simulink model "UCT_PLab"  (R2018a)
settings: Solver=VariableStepAuto  StartTime=0.0  StopTime=0.1  RelTol=1e-3
undefined symbols (not defined in the file or in its folder): DiscIntNeverNeededParam
libraries: powerlib x98
settings Model: Creator=user  LastModifiedBy=user

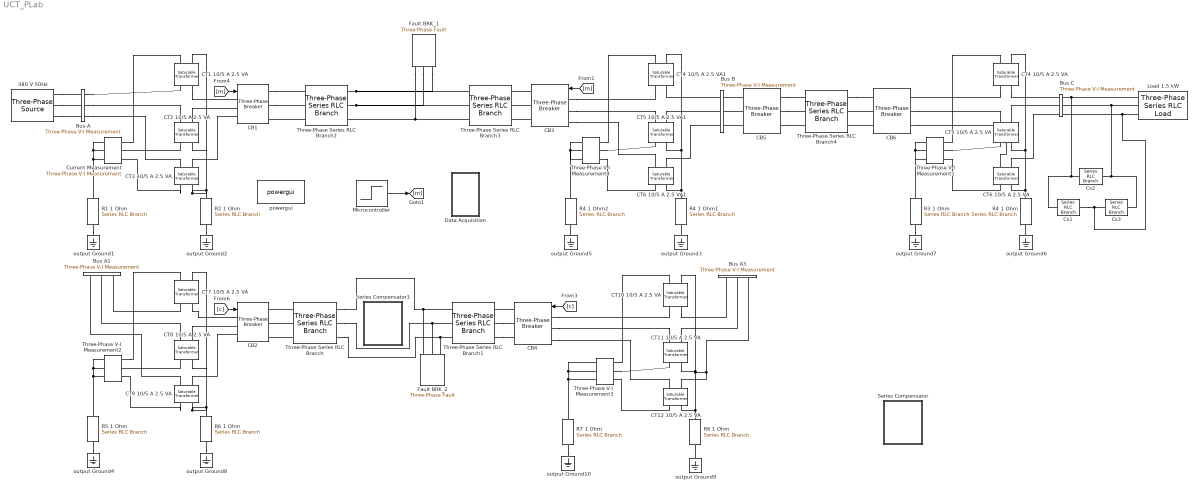
== system UCT_PLab ==
  380 V 50Hz : powerlib/Electrical Sources/Three-Phase Source  InternalConnection=Yg  VoltagePhases=off  Voltage=380  PhaseAngle=0  Voltage_phases=[25e3 25e3 25e3]/sqrt(3)  PhaseAngles_phases=[0 -120 +120]  Frequency=50  NonIdealSource=on  SpecifyImpedance=on  Resistance=132^2/30000/10  Inductance=132^2/30000/377  ShortCircuitLevel=15e3  BaseVoltage=380  XRratio=10  BusType=swing  Pref=150e6  Qref=0  Prefabc=[10e3, 10e3, 10e3]  Qrefabc=[0, 0, 0]  Qmin=0  Qmax=5e6
  Bus A : powerlib/Measurements/Three-Phase V-I Measurement  VoltageMeasurement=phase-to-phase  SetLabelV=on  LabelV=Vabc_B1  Vpu=off  VpuLL=on  CurrentMeasurement=yes  SetLabelI=on  LabelI=Iabc_B1  Ipu=off  Pbase=100e6  Vbase=380  OutputType=Complex  PhasorSimulation=off  PSBequivalent=0
  Bus A1 : powerlib/Measurements/Three-Phase V-I Measurement  VoltageMeasurement=no  SetLabelV=on  LabelV=Vabc_B1  Vpu=off  VpuLL=on  CurrentMeasurement=no  SetLabelI=on  LabelI=Iabc_B1  Ipu=off  Pbase=100e6  Vbase=380  OutputType=Complex  PhasorSimulation=off  PSBequivalent=0
  Bus A3 : powerlib/Measurements/Three-Phase V-I Measurement  VoltageMeasurement=no  SetLabelV=on  LabelV=Vabc_B1  Vpu=off  VpuLL=on  CurrentMeasurement=no  SetLabelI=on  LabelI=Iabc_B1  Ipu=off  Pbase=100e6  Vbase=380  OutputType=Complex  PhasorSimulation=off  PSBequivalent=0
  Bus B : powerlib/Measurements/Three-Phase V-I Measurement  VoltageMeasurement=phase-to-phase  SetLabelV=on  LabelV=Vabc_B2  Vpu=off  VpuLL=on  CurrentMeasurement=yes  SetLabelI=on  LabelI=Iabc_B2  Ipu=off  Pbase=100e6  Vbase=380  OutputType=Complex  PhasorSimulation=off  PSBequivalent=0
  Bus C : powerlib/Measurements/Three-Phase V-I Measurement  VoltageMeasurement=no  SetLabelV=on  LabelV=Vabc_B3  Vpu=off  VpuLL=on  CurrentMeasurement=no  SetLabelI=on  LabelI=Iabc_B3  Ipu=off  Pbase=100e6  Vbase=380  OutputType=Complex  PhasorSimulation=off  PSBequivalent=0
  CB1 : powerlib/Elements/Three-Phase Breaker  InitialState=closed  SwitchA=off  SwitchB=off  SwitchC=off  SwitchTimes=[5/60]  External=on  BreakerResistance=0.001  SnubberResistance=10e6  SnubberCapacitance=inf  Measurements=None
      settings: AttributesFormatString=\n
  CB2 : powerlib/Elements/Three-Phase Breaker  InitialState=open  SwitchA=on  SwitchB=on  SwitchC=on  SwitchTimes=[5/60]  External=on  BreakerResistance=0.001  SnubberResistance=1000e6  SnubberCapacitance=inf  Measurements=None
      settings: AttributesFormatString=\n
  CB3 : powerlib/Elements/Three-Phase Breaker  InitialState=closed  SwitchA=off  SwitchB=off  SwitchC=off  SwitchTimes=[5/60]  External=on  BreakerResistance=0.001  SnubberResistance=10e6  SnubberCapacitance=inf  Measurements=None
      settings: AttributesFormatString=\n
  CB4 : powerlib/Elements/Three-Phase Breaker  InitialState=open  SwitchA=off  SwitchB=off  SwitchC=off  SwitchTimes=[5/60]  External=on  BreakerResistance=0.001  SnubberResistance=1000e6  SnubberCapacitance=inf  Measurements=None
      settings: AttributesFormatString=\n
  CB5 : powerlib/Elements/Three-Phase Breaker  InitialState=closed  SwitchA=off  SwitchB=off  SwitchC=off  SwitchTimes=[1/60]  External=off  BreakerResistance=0.001  SnubberResistance=10e6  SnubberCapacitance=inf  Measurements=None
      settings: AttributesFormatString=\n
  CB6 : powerlib/Elements/Three-Phase Breaker  InitialState=closed  SwitchA=off  SwitchB=off  SwitchC=off  SwitchTimes=[1/60]  External=off  BreakerResistance=0.001  SnubberResistance=10e6  SnubberCapacitance=inf  Measurements=None
      settings: AttributesFormatString=\n
  CT1 10/5 A 2.5 VA : powerlib/Elements/Saturable Transformer  ThreeWindings=off  Hysteresis=off  DataFile='hysteresis'  Measurements=Winding currents  UNITS=pu  NominalPower=[2.5 50]  Winding1=[2.5*5/10 0.001 0.04]  Winding2=[5 0.001 0.04]  Winding3=[5 0.001 0.039999]  Saturation=[0 0 ; 0.01 10 ; 1 10.5]  CoreLoss=100  MoreParameters=off  BreakLoop=off  DataType=off  InitialFlux=-1.58250193491149e-05  TransfoNumber=1
      settings: AttributesFormatString=\n  SourceProductName=Simscape Power Systems  SourceProductBaseCode=PS
  CT10 10/5 A 2.5 VA : powerlib/Elements/Saturable Transformer  ThreeWindings=off  Hysteresis=off  DataFile='hysteresis'  Measurements=Winding currents  UNITS=pu  NominalPower=[15 50]  Winding1=[5*5/40 0.001 0.04]  Winding2=[5 0.001 0.04]  Winding3=[5 0.001 0.039999]  Saturation=[0 0 ; 0.01 10 ; 1 10.5]  CoreLoss=100  MoreParameters=off  BreakLoop=off  DataType=off  InitialFlux=0  TransfoNumber=1
      settings: AttributesFormatString=\n  SourceProductName=Simscape Power Systems  SourceProductBaseCode=PS
  CT11 10/5 A 2.5 VA : powerlib/Elements/Saturable Transformer  ThreeWindings=off  Hysteresis=off  DataFile='hysteresis'  Measurements=Winding currents  UNITS=pu  NominalPower=[15 50]  Winding1=[5*5/40 0.001 0.04]  Winding2=[5 0.001 0.04 ]  Winding3=[5 0.001 0.04 ]  Saturation=[0 0 ; 0.01 10 ; 1 10.5]  CoreLoss=100  MoreParameters=off  BreakLoop=off  DataType=off  InitialFlux=0  TransfoNumber=1
      settings: AttributesFormatString=\n  SourceProductName=Simscape Power Systems  SourceProductBaseCode=PS
  CT12 10/5 A 2.5 VA : powerlib/Elements/Saturable Transformer  ThreeWindings=off  Hysteresis=off  DataFile='hysteresis'  Measurements=Winding currents  UNITS=pu  NominalPower=[15 50]  Winding1=[5*5/40 0.001 0.04]  Winding2=[5 0.001 0.04]  Winding3=[5 0.001 0.039999]  Saturation=[0 0 ; 0.01 10 ; 1 10.5]  CoreLoss=100  MoreParameters=off  BreakLoop=off  DataType=off  InitialFlux=0  TransfoNumber=1
      settings: AttributesFormatString=\n  SourceProductName=Simscape Power Systems  SourceProductBaseCode=PS
  CT2 10/5 A 2.5 VA : powerlib/Elements/Saturable Transformer  ThreeWindings=off  Hysteresis=off  DataFile='hysteresis'  Measurements=Winding currents  UNITS=pu  NominalPower=[2.5 50]  Winding1=[2.5*5/10 0.001 0.04]  Winding2=[5 0.001 0.04 ]  Winding3=[5 0.001 0.04 ]  Saturation=[0 0 ; 0.01 10 ; 1 10.5]  CoreLoss=100  MoreParameters=off  BreakLoop=off  DataType=off  InitialFlux=5.84628665097414e-06  TransfoNumber=1
      settings: AttributesFormatString=\n  SourceProductName=Simscape Power Systems  SourceProductBaseCode=PS
  CT3 10/5 A 2.5 VA : powerlib/Elements/Saturable Transformer  ThreeWindings=off  Hysteresis=off  DataFile='hysteresis'  Measurements=Winding currents  UNITS=pu  NominalPower=[2.5 50]  Winding1=[2.5*5/10 0.001 0.04]  Winding2=[5 0.001 0.04]  Winding3=[5 0.001 0.039999]  Saturation=[0 0 ; 0.01 10 ; 1 10.5]  CoreLoss=100  MoreParameters=off  BreakLoop=off  DataType=off  InitialFlux=9.97873269594806e-06  TransfoNumber=1
      settings: AttributesFormatString=\n  SourceProductName=Simscape Power Systems  SourceProductBaseCode=PS
  CT4 10/5 A 2.5 VA : powerlib/Elements/Saturable Transformer  ThreeWindings=off  Hysteresis=off  DataFile='hysteresis'  Measurements=Winding currents  UNITS=pu  NominalPower=[2.5 50]  Winding1=[2.5*5/10 0.001 0.04]  Winding2=[5 0.001 0.04]  Winding3=[5 0.001 0.039999]  Saturation=[0 0 ; 0.01 10 ; 1 10.5]  CoreLoss=100  MoreParameters=off  BreakLoop=off  DataType=off  InitialFlux=-1.58243299206724e-05  TransfoNumber=1
      settings: AttributesFormatString=\n  SourceProductName=Simscape Power Systems  SourceProductBaseCode=PS
  CT4 10/5 A 2.5 VA1 : powerlib/Elements/Saturable Transformer  ThreeWindings=off  Hysteresis=off  DataFile='hysteresis'  Measurements=Winding currents  UNITS=pu  NominalPower=[2.5 50]  Winding1=[2.5*5/10 0.001 0.04]  Winding2=[5 0.001 0.04]  Winding3=[5 0.001 0.039999]  Saturation=[0 0 ; 0.01 10 ; 1 10.5]  CoreLoss=100  MoreParameters=off  BreakLoop=off  DataType=off  InitialFlux=-1.58243299202559e-05  TransfoNumber=1
      link override Model/1-D Lookup Table: NumberOfTableDimensions=1
      settings: AttributesFormatString=\n  SourceProductName=Simscape Power Systems  SourceProductBaseCode=PS
  CT5 10/5 A 2.5 VA : powerlib/Elements/Saturable Transformer  ThreeWindings=off  Hysteresis=off  DataFile='hysteresis'  Measurements=Winding currents  UNITS=pu  NominalPower=[2.5 50]  Winding1=[2.5*5/10 0.001 0.04]  Winding2=[5 0.001 0.04 ]  Winding3=[5 0.001 0.04 ]  Saturation=[0 0 ; 0.01 10 ; 1 10.5]  CoreLoss=100  MoreParameters=off  BreakLoop=off  DataType=off  InitialFlux=5.86672769127917e-06  TransfoNumber=1
      settings: AttributesFormatString=\n  SourceProductName=Simscape Power Systems  SourceProductBaseCode=PS
  CT5 10/5 A 2.5 VA1 : powerlib/Elements/Saturable Transformer  ThreeWindings=off  Hysteresis=off  DataFile='hysteresis'  Measurements=Winding currents  UNITS=pu  NominalPower=[2.5 50]  Winding1=[2.5*5/10 0.001 0.04]  Winding2=[5 0.001 0.04 ]  Winding3=[5 0.001 0.04 ]  Saturation=[0 0 ; 0.01 10 ; 1 10.5]  CoreLoss=100  MoreParameters=off  BreakLoop=off  DataType=off  InitialFlux=5.86672769116839e-06  TransfoNumber=1
      settings: AttributesFormatString=\n  SourceProductName=Simscape Power Systems  SourceProductBaseCode=PS
  CT6 10/5 A 2.5 VA : powerlib/Elements/Saturable Transformer  ThreeWindings=off  Hysteresis=off  DataFile='hysteresis'  Measurements=Winding currents  UNITS=pu  NominalPower=[2.5 50]  Winding1=[2.5*5/10 0.001 0.04]  Winding2=[5 0.001 0.04]  Winding3=[5 0.001 0.039999]  Saturation=[0 0 ; 0.01 10 ; 1 10.5]  CoreLoss=100  MoreParameters=off  BreakLoop=off  DataType=off  InitialFlux=9.95760222411303e-06  TransfoNumber=1
      settings: AttributesFormatString=\n  SourceProductName=Simscape Power Systems  SourceProductBaseCode=PS
  CT6 10/5 A 2.5 VA1 : powerlib/Elements/Saturable Transformer  ThreeWindings=off  Hysteresis=off  DataFile='hysteresis'  Measurements=Winding currents  UNITS=pu  NominalPower=[2.5 50]  Winding1=[2.5*5/10 0.001 0.04]  Winding2=[5 0.001 0.04]  Winding3=[5 0.001 0.039999]  Saturation=[0 0 ; 0.01 10 ; 1 10.5]  CoreLoss=100  MoreParameters=off  BreakLoop=off  DataType=off  InitialFlux=9.95760222411131e-06  TransfoNumber=1
      settings: AttributesFormatString=\n  SourceProductName=Simscape Power Systems  SourceProductBaseCode=PS
  CT7 10/5 A 2.5 VA : powerlib/Elements/Saturable Transformer  ThreeWindings=off  Hysteresis=off  DataFile='hysteresis'  Measurements=Winding currents  UNITS=pu  NominalPower=[15 50]  Winding1=[5*1/600 0.001 0.04]  Winding2=[5*5/40 0.001 0.04]  Winding3=[5 0.001 0.039999]  Saturation=[0 0 ; 0.01 10 ; 1 10.5]  CoreLoss=100  MoreParameters=off  BreakLoop=off  DataType=off  InitialFlux=0  TransfoNumber=1
      settings: AttributesFormatString=\n  SourceProductName=Simscape Power Systems  SourceProductBaseCode=PS
  CT8 10/5 A 2.5 VA : powerlib/Elements/Saturable Transformer  ThreeWindings=off  Hysteresis=off  DataFile='hysteresis'  Measurements=Winding currents  UNITS=pu  NominalPower=[15 50]  Winding1=[5*5/40 0.001 0.04]  Winding2=[5 0.001 0.04 ]  Winding3=[5 0.001 0.04 ]  Saturation=[0 0 ; 0.01 10 ; 1 10.5]  CoreLoss=100  MoreParameters=off  BreakLoop=off  DataType=off  InitialFlux=0  TransfoNumber=1
      settings: AttributesFormatString=\n  SourceProductName=Simscape Power Systems  SourceProductBaseCode=PS
  CT9 10/5 A 2.5 VA : powerlib/Elements/Saturable Transformer  ThreeWindings=off  Hysteresis=off  DataFile='hysteresis'  Measurements=Winding currents  UNITS=pu  NominalPower=[15 50]  Winding1=[5*5/40 0.001 0.04]  Winding2=[5 0.001 0.04]  Winding3=[5 0.001 0.039999]  Saturation=[0 0 ; 0.01 10 ; 1 10.5]  CoreLoss=100  MoreParameters=off  BreakLoop=off  DataType=off  InitialFlux=0  TransfoNumber=1
      settings: AttributesFormatString=\n  SourceProductName=Simscape Power Systems  SourceProductBaseCode=PS
  Cs1 : powerlib/Elements/Series RLC Branch  LConnTagsString=__new0  RConnTagsString=__new0  BranchType=C  Resistance=1.0  Inductance=1.0  SetiL0=off  InitialCurrent=0  Capacitance=2.0e-6  Setx0=off  InitialVoltage=0  Measurements=None
  Cs2 : powerlib/Elements/Series RLC Branch  LConnTagsString=__new0  RConnTagsString=__new0  BranchType=C  Resistance=1.0  Inductance=1.0  SetiL0=off  InitialCurrent=0  Capacitance=2.0e-6  Setx0=off  InitialVoltage=0  Measurements=None
  Cs3 : powerlib/Elements/Series RLC Branch  LConnTagsString=__new0  RConnTagsString=__new0  BranchType=C  Resistance=1.0  Inductance=1.0  SetiL0=off  InitialCurrent=0  Capacitance=2.0e-6  Setx0=off  InitialVoltage=0  Measurements=None
  Current Measurement : powerlib/Measurements/Three-Phase V-I Measurement  VoltageMeasurement=no  SetLabelV=off  LabelV=Vabc  Vpu=off  VpuLL=off  CurrentMeasurement=yes  SetLabelI=on  LabelI=Iabc  Ipu=off  Pbase=100e6  Vbase=500e3  OutputType=Complex  PhasorSimulation=off  PSBequivalent=0
  Data Acquisition : Subsystem  mask(Data Acquisition){}
      mask Display: disp('Scopes')
  Fault BRK_1 : powerlib/Elements/Three-Phase Fault  InitialStates=0  FaultA=on  FaultB=on  FaultC=on  GroundFault=on  SwitchTimes=[1/60 ]  External=off  SwitchStatus=NaN  FaultResistance=0.0001  GroundResistance=10  SnubberResistance=1e6  SnubberCapacitance=inf  Measurements=Fault currents
  Fault BRK_2 : powerlib/Elements/Three-Phase Fault  InitialStates=0  FaultA=off  FaultB=off  FaultC=off  GroundFault=off  SwitchTimes=[1/60 8/60]  External=off  SwitchStatus=NaN  FaultResistance=0.001  GroundResistance=0.01  SnubberResistance=1e6  SnubberCapacitance=inf  Measurements=Fault currents
  Load 1.5 kW : powerlib/Elements/Three-Phase Series RLC Load  LConnTagsString=A|B|C  Configuration=Y (grounded)  NominalVoltage=380  Vabc=[1e3 1e3 1e3]  Vabcp=[1e3 1e3 1e3]  NominalFrequency=50  UnbalancedPower=off  ActivePower=16.85  InductivePower=95.05  CapacitivePower=0  Pabc=[10e3 9e3 11e3]  QLabc=[100 90 110]  QCabc=[100 90 110]  Pabcp=[10e3 9e3 11e3]  QLabcp=[100 90 110]  QCabcp=[100 90 110]  Measurements=None  LoadType=constant Z
  Microcontroller : Step  Time=4/60  Before=1  VectorParams1D=off  ZeroCross=off
  R1 1 Ohm : powerlib/Elements/Series RLC Branch  LConnTagsString=__new0  RConnTagsString=__new0  BranchType=R  Resistance=1  Inductance=[]  SetiL0=off  InitialCurrent=0  Capacitance=[]  Setx0=off  InitialVoltage=0  Measurements=None
  R2 1 Ohm : powerlib/Elements/Series RLC Branch  LConnTagsString=__new0  RConnTagsString=__new0  BranchType=R  Resistance=1  Inductance=[]  SetiL0=off  InitialCurrent=0  Capacitance=[]  Setx0=off  InitialVoltage=0  Measurements=None
  R3 1 Ohm : powerlib/Elements/Series RLC Branch  LConnTagsString=__new0  RConnTagsString=__new0  BranchType=R  Resistance=1  Inductance=[]  SetiL0=off  InitialCurrent=0  Capacitance=[]  Setx0=off  InitialVoltage=0  Measurements=None
  R4 1 Ohm : powerlib/Elements/Series RLC Branch  LConnTagsString=__new0  RConnTagsString=__new0  BranchType=R  Resistance=1  Inductance=[]  SetiL0=off  InitialCurrent=0  Capacitance=[]  Setx0=off  InitialVoltage=0  Measurements=None
  R4 1 Ohm1 : powerlib/Elements/Series RLC Branch  LConnTagsString=__new0  RConnTagsString=__new0  BranchType=R  Resistance=1  Inductance=[]  SetiL0=off  InitialCurrent=0  Capacitance=[]  Setx0=off  InitialVoltage=0  Measurements=None
  R4 1 Ohm2 : powerlib/Elements/Series RLC Branch  LConnTagsString=__new0  RConnTagsString=__new0  BranchType=R  Resistance=1  Inductance=[]  SetiL0=off  InitialCurrent=0  Capacitance=[]  Setx0=off  InitialVoltage=0  Measurements=None
  R5 1 Ohm : powerlib/Elements/Series RLC Branch  LConnTagsString=__new0  RConnTagsString=__new0  BranchType=R  Resistance=1  Inductance=[]  SetiL0=off  InitialCurrent=0  Capacitance=[]  Setx0=off  InitialVoltage=0  Measurements=None
  R6 1 Ohm : powerlib/Elements/Series RLC Branch  LConnTagsString=__new0  RConnTagsString=__new0  BranchType=R  Resistance=1  Inductance=[]  SetiL0=off  InitialCurrent=0  Capacitance=[]  Setx0=off  InitialVoltage=0  Measurements=None
  R7 1 Ohm : powerlib/Elements/Series RLC Branch  LConnTagsString=__new0  RConnTagsString=__new0  BranchType=R  Resistance=1  Inductance=[]  SetiL0=off  InitialCurrent=0  Capacitance=[]  Setx0=off  InitialVoltage=0  Measurements=None
  R8 1 Ohm : powerlib/Elements/Series RLC Branch  LConnTagsString=__new0  RConnTagsString=__new0  BranchType=R  Resistance=1  Inductance=[]  SetiL0=off  InitialCurrent=0  Capacitance=[]  Setx0=off  InitialVoltage=0  Measurements=None
  Series Compensator : Subsystem
      mask Display: plot(0,0,100,100,[25 45],[50 50], [45 45],[35 65],[55 55],[35 65], [55 75],[50 50])
  Series Compensator1 : Subsystem
      mask Display: plot(0,0,100,100,[25 45],[50 50], [45 45],[35 65],[55 55],[35 65], [55 75],[50 50])
  Three-Phase Series RLC Branch : powerlib/Elements/Three-Phase Series RLC Branch  LConnTagsString=A|B|C  RConnTagsString=A|B|C  BranchType=RL  Resistance=1.60  Inductance=6.47e-3  Capacitance=0  Measurements=None
  Three-Phase Series RLC Branch1 : powerlib/Elements/Three-Phase Series RLC Branch  LConnTagsString=A|B|C  RConnTagsString=A|B|C  BranchType=RL  Resistance=1.60  Inductance=6.47e-3  Capacitance=0  Measurements=None
  Three-Phase Series RLC Branch2 : powerlib/Elements/Three-Phase Series RLC Branch  LConnTagsString=A|B|C  RConnTagsString=A|B|C  BranchType=RL  Resistance=1.60  Inductance=106.47e-3  Capacitance=0  Measurements=None
  Three-Phase Series RLC Branch3 : powerlib/Elements/Three-Phase Series RLC Branch  LConnTagsString=A|B|C  RConnTagsString=A|B|C  BranchType=RL  Resistance=1.60  Inductance=6.47e-3  Capacitance=0  Measurements=None
  Three-Phase Series RLC Branch4 : powerlib/Elements/Three-Phase Series RLC Branch  LConnTagsString=A|B|C  RConnTagsString=A|B|C  BranchType=RL  Resistance=1.35  Inductance=7.25e-3  Capacitance=0  Measurements=None
  Three-Phase V-I Measurement1 : powerlib/Measurements/Three-Phase V-I Measurement  VoltageMeasurement=no  SetLabelV=off  LabelV=Vabc  Vpu=off  VpuLL=off  CurrentMeasurement=yes  SetLabelI=on  LabelI=Iabc1  Ipu=off  Pbase=100e6  Vbase=500e3  OutputType=Complex  PhasorSimulation=off  PSBequivalent=0
  Three-Phase V-I Measurement2 : powerlib/Measurements/Three-Phase V-I Measurement  VoltageMeasurement=no  SetLabelV=off  LabelV=Vabc  Vpu=off  VpuLL=off  CurrentMeasurement=no  SetLabelI=on  LabelI=Iabc2  Ipu=off  Pbase=100e6  Vbase=500e3  OutputType=Complex  PhasorSimulation=off  PSBequivalent=0
  Three-Phase V-I Measurement3 : powerlib/Measurements/Three-Phase V-I Measurement  VoltageMeasurement=no  SetLabelV=off  LabelV=Vabc  Vpu=off  VpuLL=off  CurrentMeasurement=no  SetLabelI=on  LabelI=Iabc3  Ipu=off  Pbase=100e6  Vbase=500e3  OutputType=Complex  PhasorSimulation=off  PSBequivalent=0
  Three-Phase V-I Measurement4 : powerlib/Measurements/Three-Phase V-I Measurement  VoltageMeasurement=no  SetLabelV=off  LabelV=Vabc  Vpu=off  VpuLL=off  CurrentMeasurement=no  SetLabelI=on  LabelI=Iabc1  Ipu=off  Pbase=100e6  Vbase=500e3  OutputType=Complex  PhasorSimulation=off  PSBequivalent=0
  output Ground{1..10} (10 alike) : powerlib/Elements/Ground  LConnTagsString=a
  powergui : powerlib/powergui  Priority=2  SimulationMode=Discrete  SampleTime=50e-6  frequency=60  Iterations=50  frequencyindice=50  Pbase=100e6  ErrMax=0.0001  UnitsV=kV  UnitsW=MW  buscounter=0  FunctionMessages=off  echomessages=off  EnableUseOfTLC=off  CurrentSourceSwitches=off  DisableSnubberDevices=off  DisableRonSwitches=off  DisableVfSwitches=off  DisplayEquations=off  SolverType=Tustin/Backward Euler (TBE)  Interpol=off  ExternalGateDelay=off  methode=off  Ts=100  x0status=blocks  SPID=off  SwTol=0  HookPort=off  RestoreLinks=warning  ResistiveCurrentMeasurement=off  Frange=0:0.5:500  Ylog=off  Xlog=off  ShowGrid=off  save=on  variable=Zmes  structure=0  ZoomFFT=on  StartTime=0.0  cycles=1  DisplayStyle=off  fundamental=60  FreqAxis=off  MaxFrequency=1000  frequencyindicesteady=1  RmsSteady=1  display=off
  wires:
  Microcontroller/1 -> [m]
  [m] -> CB3/1
  [m] -> CB1/1
  [c] -> CB4/1
  [c] -> CB2/1
  connections:
  CT9 10/5 A 2.5 VA/LConn1 -- Bus A1/RConn3
  Bus A/RConn1 -- CT1 10/5 A 2.5 VA/LConn1
  Current Measurement/RConn3 -- R1 1 Ohm/LConn1 -- Current Measurement/RConn2 -- Current Measurement/RConn1
  Bus A/RConn2 -- CT2 10/5 A 2.5 VA/LConn1
  CT3 10/5 A 2.5 VA/RConn2 -- R2 1 Ohm/LConn1 -- CT1 10/5 A 2.5 VA/RConn2 -- CT2 10/5 A 2.5 VA/RConn2
  380 V 50Hz/RConn1 -- Bus A/LConn1
  380 V 50Hz/RConn3 -- Bus A/LConn3
  CB3/RConn3 -- Three-Phase Series RLC Branch3/RConn3
  CB1/RConn1 -- Three-Phase Series RLC Branch2/LConn1
  CB1/RConn2 -- Three-Phase Series RLC Branch2/LConn2
  CT3 10/5 A 2.5 VA/RConn1 -- Current Measurement/LConn3
  CB3/RConn2 -- Three-Phase Series RLC Branch3/RConn2
  CB3/RConn1 -- Three-Phase Series RLC Branch3/RConn1
  CT2 10/5 A 2.5 VA/LConn2 -- CB1/LConn2
  CB1/LConn3 -- CT3 10/5 A 2.5 VA/LConn2
  380 V 50Hz/RConn2 -- Bus A/LConn2
  CT1 10/5 A 2.5 VA/LConn2 -- CB1/LConn1
  Current Measurement/LConn1 -- CT1 10/5 A 2.5 VA/RConn1
  R2 1 Ohm/RConn1 -- output Ground2/LConn1
  R1 1 Ohm/RConn1 -- output Ground1/LConn1
  CT2 10/5 A 2.5 VA/RConn1 -- Current Measurement/LConn2
  CT9 10/5 A 2.5 VA/RConn2 -- R6 1 Ohm/LConn1 -- CT7 10/5 A 2.5 VA/RConn2 -- CT8 10/5 A 2.5 VA/RConn2
  Three-Phase V-I Measurement2/RConn3 -- Three-Phase V-I Measurement2/RConn1 -- Three-Phase V-I Measurement2/RConn2 -- R5 1 Ohm/LConn1
  Three-Phase Series RLC Branch/RConn1 -- Three-Phase Series RLC Branch1/LConn1 -- Fault BRK_2/LConn1
  Three-Phase Series RLC Branch/RConn2 -- Three-Phase Series RLC Branch1/LConn2 -- Fault BRK_2/LConn2
  Three-Phase Series RLC Branch/RConn3 -- Three-Phase Series RLC Branch1/LConn3 -- Fault BRK_2/LConn3
  R7 1 Ohm/LConn1 -- Three-Phase V-I Measurement3/RConn3 -- Three-Phase V-I Measurement3/RConn2 -- Three-Phase V-I Measurement3/RConn1
  Three-Phase Series RLC Branch1/RConn2 -- CB4/RConn2
  R5 1 Ohm/RConn1 -- output Ground4/LConn1
  CT8 10/5 A 2.5 VA/RConn1 -- Three-Phase V-I Measurement2/LConn2
  CT9 10/5 A 2.5 VA/RConn1 -- Three-Phase V-I Measurement2/LConn3
  CB4/LConn3 -- CT12 10/5 A 2.5 VA/LConn1
  CT7 10/5 A 2.5 VA/LConn2 -- CB2/LConn1
  CB2/LConn3 -- CT9 10/5 A 2.5 VA/LConn2
  output Ground9/LConn1 -- R8 1 Ohm/RConn1
  Three-Phase Series RLC Branch1/RConn3 -- CB4/RConn3
  R7 1 Ohm/RConn1 -- output Ground10/LConn1
  CT8 10/5 A 2.5 VA/LConn2 -- CB2/LConn2
  Three-Phase V-I Measurement2/LConn1 -- CT7 10/5 A 2.5 VA/RConn1
  Three-Phase Series RLC Branch/LConn1 -- CB2/RConn1
  R6 1 Ohm/RConn1 -- output Ground8/LConn1
  Three-Phase V-I Measurement3/LConn2 -- CT11 10/5 A 2.5 VA/RConn1
  Three-Phase Series RLC Branch/LConn2 -- CB2/RConn2
  Three-Phase Series RLC Branch/LConn3 -- CB2/RConn3
  CB4/RConn1 -- Three-Phase Series RLC Branch1/RConn1
  CB4/LConn2 -- CT11 10/5 A 2.5 VA/LConn1
  Three-Phase V-I Measurement3/LConn1 -- CT10 10/5 A 2.5 VA/RConn1
  CB4/LConn1 -- CT10 10/5 A 2.5 VA/LConn1
  Three-Phase V-I Measurement3/LConn3 -- CT12 10/5 A 2.5 VA/RConn1
  CB6/RConn2 -- Three-Phase Series RLC Branch4/RConn2
  CB6/RConn3 -- Three-Phase Series RLC Branch4/RConn3
  Three-Phase Series RLC Branch4/RConn1 -- CB6/RConn1
  Cs1/RConn1 -- Bus C/RConn3 -- Load 1.5 kW/LConn3 -- Cs3/LConn1
  CB5/RConn3 -- Bus B/RConn3
  CB5/RConn1 -- Bus B/RConn1
  CB5/RConn2 -- Bus B/RConn2
  Three-Phase Series RLC Branch2/LConn3 -- CB1/RConn3
  CT8 10/5 A 2.5 VA/LConn1 -- Bus A1/RConn2
  CT7 10/5 A 2.5 VA/LConn1 -- Bus A1/RConn1
  CT11 10/5 A 2.5 VA/LConn2 -- Bus A3/RConn2
  CT10 10/5 A 2.5 VA/LConn2 -- Bus A3/RConn3
  CT11 10/5 A 2.5 VA/RConn2 -- Bus A3/RConn1 -- CT12 10/5 A 2.5 VA/LConn2 -- CT12 10/5 A 2.5 VA/RConn2 -- R8 1 Ohm/LConn1 -- CT10 10/5 A 2.5 VA/RConn2
  CB5/LConn3 -- Three-Phase Series RLC Branch4/LConn3
  CB5/LConn2 -- Three-Phase Series RLC Branch4/LConn2
  CB5/LConn1 -- Three-Phase Series RLC Branch4/LConn1
  Three-Phase Series RLC Branch2/RConn1 -- Three-Phase Series RLC Branch3/LConn1 -- Fault BRK_1/LConn1
  Three-Phase V-I Measurement1/RConn2 -- Three-Phase V-I Measurement1/RConn1 -- Three-Phase V-I Measurement1/RConn3 -- R3 1 Ohm/LConn1
  CT4 10/5 A 2.5 VA/RConn2 -- CT5 10/5 A 2.5 VA/RConn2 -- CT6 10/5 A 2.5 VA/RConn2 -- R4 1 Ohm/LConn1
  R3 1 Ohm/RConn1 -- output Ground7/LConn1
  Three-Phase V-I Measurement1/LConn2 -- CT5 10/5 A 2.5 VA/RConn1
  output Ground6/LConn1 -- R4 1 Ohm/RConn1
  CT5 10/5 A 2.5 VA/LConn2 -- Bus C/LConn2
  CB6/LConn2 -- CT5 10/5 A 2.5 VA/LConn1
  CT4 10/5 A 2.5 VA/LConn1 -- CB6/LConn1
  Three-Phase V-I Measurement1/LConn1 -- CT4 10/5 A 2.5 VA/RConn1
  CT4 10/5 A 2.5 VA/LConn2 -- Bus C/LConn1
  CB6/LConn3 -- CT6 10/5 A 2.5 VA/LConn1
  CT6 10/5 A 2.5 VA/LConn2 -- Bus C/LConn3
  Three-Phase V-I Measurement1/LConn3 -- CT6 10/5 A 2.5 VA/RConn1
  Three-Phase V-I Measurement4/RConn2 -- Three-Phase V-I Measurement4/RConn1 -- Three-Phase V-I Measurement4/RConn3 -- R4 1 Ohm2/LConn1
  CT4 10/5 A 2.5 VA1/RConn2 -- CT5 10/5 A 2.5 VA1/RConn2 -- CT6 10/5 A 2.5 VA1/RConn2 -- R4 1 Ohm1/LConn1
  CB3/LConn1 -- CT4 10/5 A 2.5 VA1/LConn1
  output Ground3/LConn1 -- R4 1 Ohm1/RConn1
  Three-Phase V-I Measurement4/LConn1 -- CT4 10/5 A 2.5 VA1/RConn1
  Three-Phase V-I Measurement4/LConn3 -- CT6 10/5 A 2.5 VA1/RConn1
  CT6 10/5 A 2.5 VA1/LConn2 -- Bus B/LConn3
  CB3/LConn3 -- CT6 10/5 A 2.5 VA1/LConn1
  Bus B/LConn1 -- CT4 10/5 A 2.5 VA1/LConn2
  Three-Phase V-I Measurement4/LConn2 -- CT5 10/5 A 2.5 VA1/RConn1
  Bus B/LConn2 -- CT5 10/5 A 2.5 VA1/LConn2
  output Ground5/LConn1 -- R4 1 Ohm2/RConn1
  CB3/LConn2 -- CT5 10/5 A 2.5 VA1/LConn1
  Bus A/RConn3 -- CT3 10/5 A 2.5 VA/LConn1
  Three-Phase Series RLC Branch2/RConn2 -- Three-Phase Series RLC Branch3/LConn2 -- Fault BRK_1/LConn2
  Fault BRK_1/LConn3 -- Three-Phase Series RLC Branch3/LConn3 -- Three-Phase Series RLC Branch2/RConn3
  Bus C/RConn2 -- Cs2/RConn1 -- Cs3/RConn1 -- Load 1.5 kW/LConn2
  Bus C/RConn1 -- Cs1/LConn1 -- Cs2/LConn1 -- Load 1.5 kW/LConn1

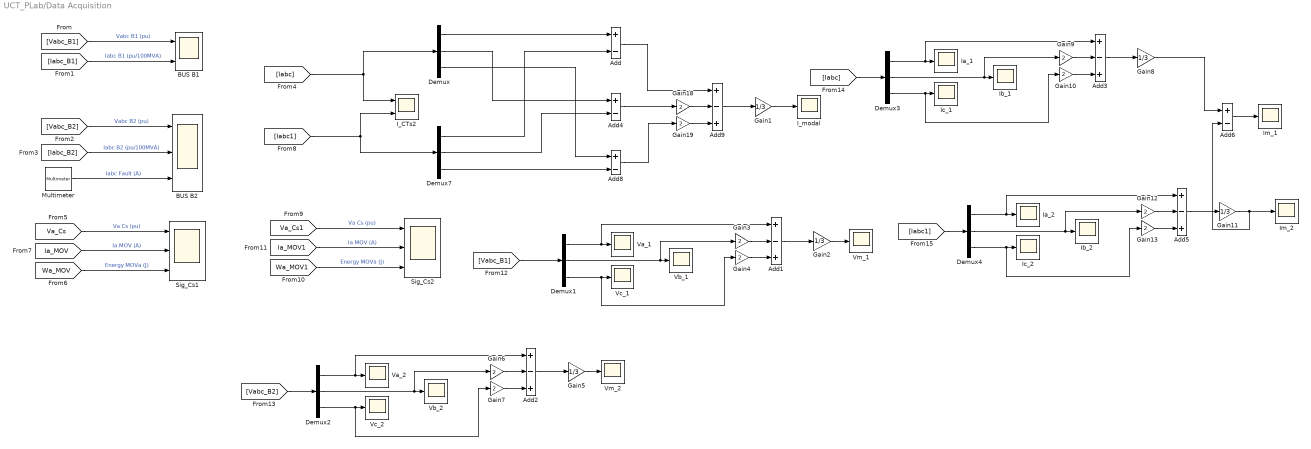
== system UCT_PLab/Data Acquisition ==
  Add{,4,6,8} (4 alike) : Sum  Inputs=+-
  Add{1..3,5,9} (5 alike) : Sum  Inputs=+-+
  BUS B1 : Scope  NumInputPorts=2
  BUS B2 : Scope  NumInputPorts=3
  Demux{,1..4,7} (6 alike) : Demux  Outputs=3
  Gain{1..2,5,8,11} (5 alike) : Gain  Gain=1/3
  Gain{3..4,6..7,9..10,12..13,18..19} (10 alike) : Gain  Gain=2
  I_CTs2 : Scope  NumInputPorts=2
  I_modal : Scope
  Ia_1 : Scope
  Ia_2 : Scope
  Ib_1 : Scope
  Ib_2 : Scope
  Ic_1 : Scope
  Ic_2 : Scope
  Im_1 : Scope
  Im_2 : Scope
  Multimeter : powerlib/Measurements/Multimeter  Tag=PoWeRsYsTeMmEaSuReMeNt  PhasorSimulation=off  OutputType=Magnitude  sel=1  L=36  Gain=0  yselected={}  PSBOutputType=1  PSBequivalent=0  AxesSetting=[0,0.1,-100,100]  Display=0  SavedBlockNames={}
      settings: AttributesFormatString=\n
  Sig_Cs1 : Scope  NumInputPorts=3
  Sig_Cs2 : Scope  NumInputPorts=3
  Va_1 : Scope
  Va_2 : Scope
  Vb_1 : Scope
  Vb_2 : Scope
  Vc_1 : Scope
  Vc_2 : Scope
  Vm_1 : Scope
  Vm_2 : Scope
  wires:
  [Vabc_B1] -> BUS B1/1  "Vabc B1 (pu)"
  [Iabc_B1] -> BUS B1/2  "Iabc B1 (pu/100MVA)"
  [Vabc_B2] -> BUS B2/1  "Vabc B2 (pu)"
  [Iabc_B2] -> BUS B2/2  "Iabc B2 (pu/100MVA)"
  [Va_Cs] -> Sig_Cs1/1  "Va Cs (pu)"
  [Ia_MOV] -> Sig_Cs1/2  "Ia MOV (A)"
  [Wa_MOV] -> Sig_Cs1/3  "Energy MOVa (J)"
  Multimeter/1 -> BUS B2/3  "Iabc Fault (A)"
  [Wa_MOV1] -> Sig_Cs2/3  "Energy MOVa (J)"
  [Ia_MOV1] -> Sig_Cs2/2  "Ia MOV (A)"
  [Va_Cs1] -> Sig_Cs2/1  "Va Cs (pu)"
  Demux/1 -> Add/1
  Demux7/1 -> Add/2
  Demux/2 -> Add4/1
  Demux7/2 -> Add4/2
  Demux7/3 -> Add8/2
  Demux/3 -> Add8/1
  Add8/1 -> Gain19/1
  Gain18/1 -> Add9/2
  Gain19/1 -> Add9/3
  Add9/1 -> Gain1/1
  Add/1 -> Add9/1
  Add4/1 -> Gain18/1
  [Iabc1] -> I_CTs2/2, Demux7/1
  [Iabc] -> Demux/1, I_CTs2/1
  [Vabc_B1] -> Demux1/1
  Demux1/2 -> Gain3/1, Vb_1/1
  Demux1/3 -> Gain4/1, Vc_1/1
  Demux1/1 -> Add1/1, Va_1/1
  Gain3/1 -> Add1/2
  Gain4/1 -> Add1/3
  Add1/1 -> Gain2/1
  Demux2/1 -> Add2/1, Va_2/1
  Demux2/3 -> Gain7/1, Vc_2/1
  [Vabc_B2] -> Demux2/1
  Demux2/2 -> Gain6/1, Vb_2/1
  Gain7/1 -> Add2/3
  Gain6/1 -> Add2/2
  Gain5/1 -> Vm_2/1
  Add2/1 -> Gain5/1
  Gain2/1 -> Vm_1/1
  Gain1/1 -> I_modal/1
  Demux3/1 -> Add3/1, Ia_1/1
  Demux3/3 -> Gain10/1, Ic_1/1
  [Iabc] -> Demux3/1
  Demux3/2 -> Gain9/1, Ib_1/1
  Gain9/1 -> Add3/2
  Add3/1 -> Gain8/1
  Gain10/1 -> Add3/3
  Demux4/1 -> Add5/1, Ia_2/1
  Demux4/3 -> Gain13/1, Ic_2/1
  [Iabc1] -> Demux4/1
  Gain11/1 -> Add6/2, Im_2/1
  Demux4/2 -> Gain12/1, Ib_2/1
  Gain12/1 -> Add5/2
  Add5/1 -> Gain11/1
  Gain13/1 -> Add5/3
  Gain8/1 -> Add6/1
  Add6/1 -> Im_1/1

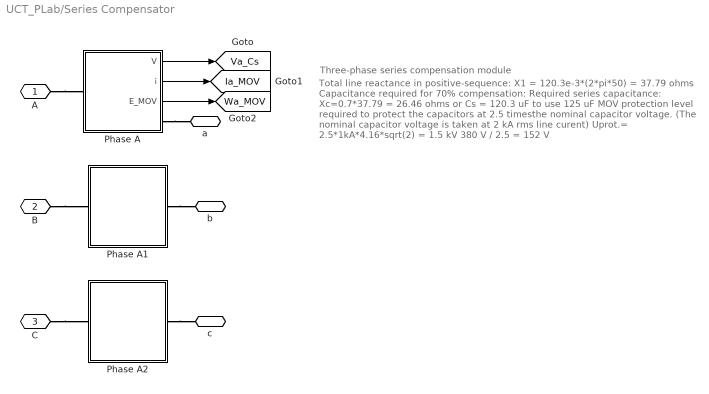
== system UCT_PLab/Series Compensator ==
  note: Three-phase series compensation module
  note: Total line reactance in positive-sequence:
      |  X1 = 120.3e-3*(2*pi*50) = 37.79 ohms
      |
      | Capacitance required for 70% compensation:
      |
      | Required series capacitance:
      | Xc=0.7*37.79 = 26.46 ohms
      | or Cs = 120.3 uF to use 125 uF
      |
      | MOV protection level required to protect the capacitors
      | at 2.5 timesthe nominal capacitor voltage.
      | (The nominal capacitor voltage is taken at 2 kA  rms line curent)
      |
      | Uprot.= 2.5*1kA*4.16*sqrt(2) = 1.5 kV
      |
      | 380 V / 2.5 = 152 V
  Phase A : Subsystem
  Phase A1 : Subsystem
  Phase A2 : Subsystem
  A : PMIOPort  Side=Left
  B : PMIOPort  Port=2  Side=Left
  C : PMIOPort  Port=3  Side=Left
  a : PMIOPort  Port=4  Side=Right
  b : PMIOPort  Port=5  Side=Right
  c : PMIOPort  Port=6  Side=Right
  tag scope: Ia_MOV=global, Va_Cs=global, Wa_MOV=global
  wires:
  Phase A/2(i) -> [Ia_MOV]
  Phase A/1(V) -> [Va_Cs]
  Phase A/3(E_MOV) -> [Wa_MOV]
  connections:
  A/RConn1 -- Phase A/LConn1
  B/RConn1 -- Phase A1/LConn1
  C/RConn1 -- Phase A2/LConn1
  Phase A/RConn1 -- a/RConn1
  Phase A1/RConn1 -- b/RConn1
  Phase A2/RConn1 -- c/RConn1

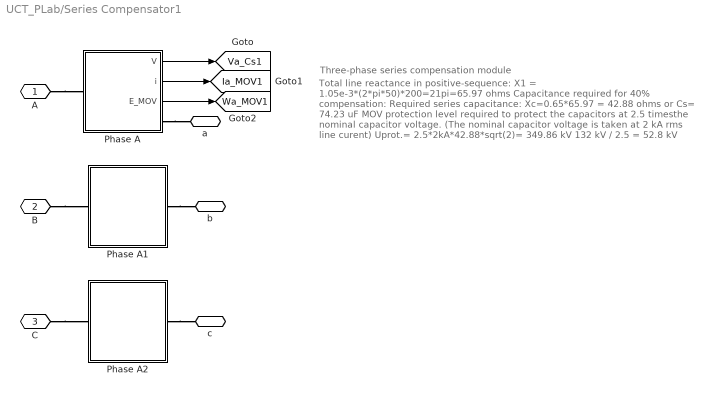
== system UCT_PLab/Series Compensator1 ==
  note: Three-phase series compensation module
  note: Total line reactance in positive-sequence:
      |  X1 = 1.05e-3*(2*pi*50)*200=21pi=65.97 ohms
      |
      | Capacitance required for 40% compensation:
      |
      | Required series capacitance:
      | Xc=0.65*65.97 = 42.88 ohms
      | or Cs= 74.23 uF
      |
      | MOV protection level required to protect the capacitors
      | at 2.5 timesthe nominal capacitor voltage.
      | (The nominal capacitor voltage is taken at 2 kA  rms line curent)
      |
      | Uprot.= 2.5*2kA*42.88*sqrt(2)= 349.86 kV
      |
      | 132 kV / 2.5 = 52.8 kV
  Phase A : Subsystem
  Phase A1 : Subsystem
  Phase A2 : Subsystem
  A : PMIOPort  Side=Left
  B : PMIOPort  Port=2  Side=Left
  C : PMIOPort  Port=3  Side=Left
  a : PMIOPort  Port=4  Side=Right
  b : PMIOPort  Port=5  Side=Right
  c : PMIOPort  Port=6  Side=Right
  tag scope: Ia_MOV1=global, Va_Cs1=global, Wa_MOV1=global
  wires:
  Phase A/2(i) -> [Ia_MOV1]
  Phase A/1(V) -> [Va_Cs1]
  Phase A/3(E_MOV) -> [Wa_MOV1]
  connections:
  A/RConn1 -- Phase A/LConn1
  B/RConn1 -- Phase A1/LConn1
  C/RConn1 -- Phase A2/LConn1
  Phase A/RConn1 -- a/RConn1
  Phase A1/RConn1 -- b/RConn1
  Phase A2/RConn1 -- c/RConn1

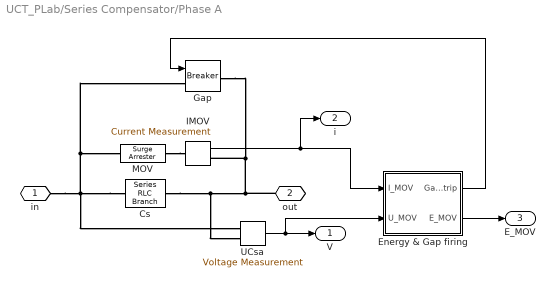
== system UCT_PLab/Series Compensator/Phase A ==
  Cs : powerlib/Elements/Series RLC Branch  LConnTagsString=__new0  RConnTagsString=__new0  BranchType=C  Resistance=1.0  Inductance=1.0  SetiL0=off  InitialCurrent=0  Capacitance=125e-6  Setx0=off  InitialVoltage=0  Measurements=None
  Energy & Gap firing : Subsystem
  Gap : powerlib/Elements/Breaker  InitialState=0  SwitchingTimes="[ 4/60  5/60 ]"  External=on  BreakerResistance=0.001  SnubberResistance=inf  SnubberCapacitance=0  Measurements=None  MoreParameters=off  NoBreakLoop=off
      settings: AttributesFormatString=\n  SourceProductName=Simscape Power Systems
  IMOV : powerlib/Measurements/Current Measurement  Tag=PoWeRsYsTeMmEaSuReMeNt  PhasorSimulation=off  OutputType=Magnitude  PSBequivalent=0
  MOV : powerlib/Elements/Surge Arrester  ProtectionVoltage=152  Columns=30  ReferenceCurrent=50  Segment1=[.955 50]  Segment2=[1.0 25]  Segment3=[.9915 16.5]  Measurements=None  BreakLoop=on
      settings: AttributesFormatString=\n  SourceProductName=Simscape Power Systems  SourceProductBaseCode=PS
  UCsa : powerlib/Measurements/Voltage Measurement  Tag=PoWeRsYsTeMmEaSuReMeNt  PhasorSimulation=off  OutputType=Magnitude  PSBequivalent=0
  in : PMIOPort  Side=Left
  "out " : PMIOPort  Port=2  Side=Right
  V : Outport
  i : Outport  Port=2
  E_MOV : Outport  Port=3
  wires:
  Energy & Gap firing/2(E_MOV) -> E_MOV/1
  IMOV/1 -> Energy & Gap firing/1(I_MOV), i/1
  UCsa/1 -> Energy & Gap firing/2(U_MOV), V/1
  Energy & Gap firing/1(Gap_trip) -> Gap/1
  connections:
  MOV/RConn1 -- IMOV/LConn1
  Cs/LConn1 -- in/RConn1 -- UCsa/LConn1 -- Gap/LConn1 -- MOV/LConn1
  Cs/RConn1 -- "out "/RConn1 -- Gap/RConn1 -- IMOV/RConn1 -- UCsa/LConn2

== system UCT_PLab/Series Compensator/Phase A1 ==
  Cs : powerlib/Elements/Series RLC Branch  LConnTagsString=__new0  RConnTagsString=__new0  BranchType=C  Resistance=1.0  Inductance=1.0  SetiL0=off  InitialCurrent=0  Capacitance=125e-6  Setx0=off  InitialVoltage=0  Measurements=None
  Energy & Gap firing : Subsystem
  Gap : powerlib/Elements/Breaker  InitialState=0  SwitchingTimes="[ 4/60  5/60 ]"  External=on  BreakerResistance=0.001  SnubberResistance=inf  SnubberCapacitance=0  Measurements=None  MoreParameters=off  NoBreakLoop=off
      settings: AttributesFormatString=\n  SourceProductName=Simscape Power Systems
  IMOV : powerlib/Measurements/Current Measurement  Tag=PoWeRsYsTeMmEaSuReMeNt  PhasorSimulation=off  OutputType=Magnitude  PSBequivalent=0
  MOV_ : powerlib/Elements/Surge Arrester  ProtectionVoltage=152  Columns=30  ReferenceCurrent=50  Segment1=[.955 50]  Segment2=[1.0 25]  Segment3=[.9915 16.5]  Measurements=None  BreakLoop=on
      settings: AttributesFormatString=\n  SourceProductName=Simscape Power Systems  SourceProductBaseCode=PS
  UCsa : powerlib/Measurements/Voltage Measurement  Tag=PoWeRsYsTeMmEaSuReMeNt  PhasorSimulation=off  OutputType=Magnitude  PSBequivalent=0
  in_ : PMIOPort  Side=Left
  "out_ " : PMIOPort  Port=2  Side=Right
  wires:
  Energy & Gap firing/1(Gap_trip) -> Gap/1
  UCsa/1 -> Energy & Gap firing/2(U_MOV)
  IMOV/1 -> Energy & Gap firing/1(I_MOV)
  connections:
  "out_ "/RConn1 -- Cs/RConn1 -- UCsa/LConn2 -- Gap/RConn1 -- IMOV/RConn1
  in_/RConn1 -- UCsa/LConn1 -- Cs/LConn1 -- Gap/LConn1 -- MOV_/LConn1
  MOV_/RConn1 -- IMOV/LConn1

== system UCT_PLab/Series Compensator/Phase A2 ==
  Cs : powerlib/Elements/Series RLC Branch  LConnTagsString=__new0  RConnTagsString=__new0  BranchType=C  Resistance=1.0  Inductance=1.0  SetiL0=off  InitialCurrent=0  Capacitance=125e-6  Setx0=off  InitialVoltage=0  Measurements=None
  Energy & Gap firing : Subsystem
  Gap : powerlib/Elements/Breaker  InitialState=0  SwitchingTimes="[ 4/60  5/60 ]"  External=on  BreakerResistance=0.001  SnubberResistance=inf  SnubberCapacitance=0  Measurements=None  MoreParameters=off  NoBreakLoop=off
      settings: AttributesFormatString=\n  SourceProductName=Simscape Power Systems
  IMOV : powerlib/Measurements/Current Measurement  Tag=PoWeRsYsTeMmEaSuReMeNt  PhasorSimulation=off  OutputType=Magnitude  PSBequivalent=0
  MOV : powerlib/Elements/Surge Arrester  ProtectionVoltage=152  Columns=30  ReferenceCurrent=50  Segment1=[.955 50]  Segment2=[1.0 25]  Segment3=[.9915 16.5]  Measurements=None  BreakLoop=on
      settings: AttributesFormatString=\n  SourceProductName=Simscape Power Systems  SourceProductBaseCode=PS
  UCsa : powerlib/Measurements/Voltage Measurement  Tag=PoWeRsYsTeMmEaSuReMeNt  PhasorSimulation=off  OutputType=Magnitude  PSBequivalent=0
  in : PMIOPort  Side=Left
  "out " : PMIOPort  Port=2  Side=Right
  wires:
  IMOV/1 -> Energy & Gap firing/1(I_MOV)
  UCsa/1 -> Energy & Gap firing/2(U_MOV)
  Energy & Gap firing/1(Gap_trip) -> Gap/1
  connections:
  MOV/RConn1 -- IMOV/LConn1
  MOV/LConn1 -- Gap/LConn1 -- in/RConn1 -- Cs/LConn1 -- UCsa/LConn1
  IMOV/RConn1 -- Gap/RConn1 -- Cs/RConn1 -- UCsa/LConn2 -- "out "/RConn1

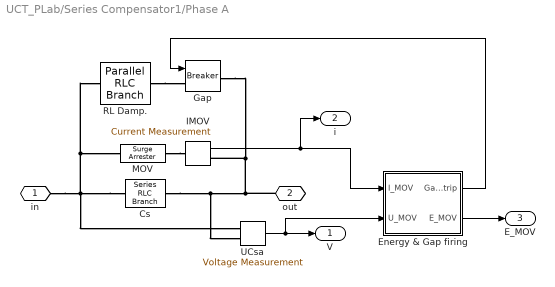
== system UCT_PLab/Series Compensator1/Phase A ==
  Cs : powerlib/Elements/Series RLC Branch  LConnTagsString=__new0  RConnTagsString=__new0  BranchType=C  Resistance=1.0  Inductance=1.0  SetiL0=off  InitialCurrent=0  Capacitance=500e-6  Setx0=off  InitialVoltage=0  Measurements=None
  Energy & Gap firing : Subsystem
  Gap : powerlib/Elements/Breaker  InitialState=0  SwitchingTimes="[ 4/60  5/60 ]"  External=on  BreakerResistance=0.001  SnubberResistance=inf  SnubberCapacitance=0  Measurements=None  MoreParameters=off  NoBreakLoop=off
      settings: AttributesFormatString=\n  SourceProductName=Simscape Power Systems
  IMOV : powerlib/Measurements/Current Measurement  Tag=PoWeRsYsTeMmEaSuReMeNt  PhasorSimulation=off  OutputType=Magnitude  PSBequivalent=0
  MOV : powerlib/Elements/Surge Arrester  ProtectionVoltage=54e+03  Columns=27  ReferenceCurrent=200  Segment1=[.955 50]  Segment2=[1.0 25]  Segment3=[.9915 16.5]  Measurements=None  BreakLoop=on
      settings: AttributesFormatString=\n  SourceProductName=Simscape Power Systems  SourceProductBaseCode=PS
  RL Damp. : powerlib/Elements/Parallel RLC Branch  LConnTagsString=a  RConnTagsString=__new0  BranchType=RL  Resistance=7.5  Inductance=1.7e-3  SetiL0=off  InitialCurrent=0  Capacitance=1.0  Setx0=off  InitialVoltage=0  Measurements=None
  UCsa : powerlib/Measurements/Voltage Measurement  Tag=PoWeRsYsTeMmEaSuReMeNt  PhasorSimulation=off  OutputType=Magnitude  PSBequivalent=0
  in : PMIOPort  Side=Left
  "out " : PMIOPort  Port=2  Side=Right
  V : Outport
  i : Outport  Port=2
  E_MOV : Outport  Port=3
  wires:
  Energy & Gap firing/2(E_MOV) -> E_MOV/1
  IMOV/1 -> Energy & Gap firing/1(I_MOV), i/1
  UCsa/1 -> Energy & Gap firing/2(U_MOV), V/1
  Energy & Gap firing/1(Gap_trip) -> Gap/1
  connections:
  MOV/RConn1 -- IMOV/LConn1
  Cs/LConn1 -- UCsa/LConn1 -- in/RConn1 -- RL Damp./LConn1 -- MOV/LConn1
  RL Damp./RConn1 -- Gap/LConn1
  Cs/RConn1 -- "out "/RConn1 -- IMOV/RConn1 -- Gap/RConn1 -- UCsa/LConn2

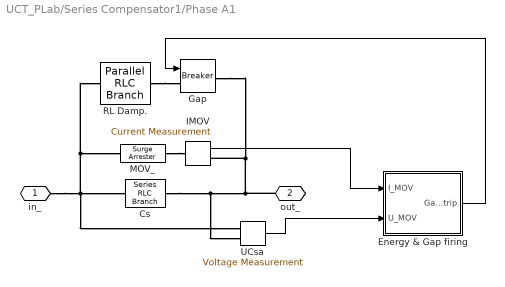
== system UCT_PLab/Series Compensator1/Phase A1 ==
  Cs : powerlib/Elements/Series RLC Branch  LConnTagsString=__new0  RConnTagsString=__new0  BranchType=C  Resistance=1.0  Inductance=1.0  SetiL0=off  InitialCurrent=0  Capacitance=500e-6  Setx0=off  InitialVoltage=0  Measurements=None
  Energy & Gap firing : Subsystem
  Gap : powerlib/Elements/Breaker  InitialState=0  SwitchingTimes="[ 4/60  5/60 ]"  External=on  BreakerResistance=0.001  SnubberResistance=inf  SnubberCapacitance=0  Measurements=None  MoreParameters=off  NoBreakLoop=off
      settings: AttributesFormatString=\n  SourceProductName=Simscape Power Systems
  IMOV : powerlib/Measurements/Current Measurement  Tag=PoWeRsYsTeMmEaSuReMeNt  PhasorSimulation=off  OutputType=Magnitude  PSBequivalent=0
  MOV_ : powerlib/Elements/Surge Arrester  ProtectionVoltage=54e+03  Columns=27  ReferenceCurrent=200  Segment1=[.955 50]  Segment2=[1.0 25]  Segment3=[.9915 16.5]  Measurements=None  BreakLoop=on
      settings: AttributesFormatString=\n  SourceProductName=Simscape Power Systems  SourceProductBaseCode=PS
  RL Damp. : powerlib/Elements/Parallel RLC Branch  LConnTagsString=a  RConnTagsString=__new0  BranchType=RL  Resistance=7.5  Inductance=1.7e-3  SetiL0=off  InitialCurrent=0  Capacitance=1.0  Setx0=off  InitialVoltage=0  Measurements=None
  UCsa : powerlib/Measurements/Voltage Measurement  Tag=PoWeRsYsTeMmEaSuReMeNt  PhasorSimulation=off  OutputType=Magnitude  PSBequivalent=0
  in_ : PMIOPort  Side=Left
  "out_ " : PMIOPort  Port=2  Side=Right
  wires:
  Energy & Gap firing/1(Gap_trip) -> Gap/1
  UCsa/1 -> Energy & Gap firing/2(U_MOV)
  IMOV/1 -> Energy & Gap firing/1(I_MOV)
  connections:
  "out_ "/RConn1 -- UCsa/LConn2 -- Cs/RConn1 -- Gap/RConn1 -- IMOV/RConn1
  RL Damp./RConn1 -- Gap/LConn1
  in_/RConn1 -- UCsa/LConn1 -- Cs/LConn1 -- MOV_/LConn1 -- RL Damp./LConn1
  MOV_/RConn1 -- IMOV/LConn1

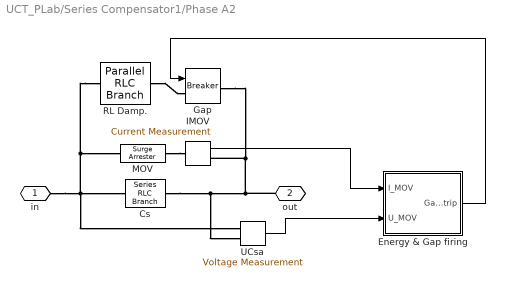
== system UCT_PLab/Series Compensator1/Phase A2 ==
  Cs : powerlib/Elements/Series RLC Branch  LConnTagsString=__new0  RConnTagsString=__new0  BranchType=C  Resistance=1.0  Inductance=1.0  SetiL0=off  InitialCurrent=0  Capacitance=500e-6  Setx0=off  InitialVoltage=0  Measurements=None
  Energy & Gap firing : Subsystem
  Gap : powerlib/Elements/Breaker  InitialState=0  SwitchingTimes="[ 4/60  5/60 ]"  External=on  BreakerResistance=0.001  SnubberResistance=inf  SnubberCapacitance=0  Measurements=None  MoreParameters=off  NoBreakLoop=off
      settings: AttributesFormatString=\n  SourceProductName=Simscape Power Systems
  IMOV : powerlib/Measurements/Current Measurement  Tag=PoWeRsYsTeMmEaSuReMeNt  PhasorSimulation=off  OutputType=Magnitude  PSBequivalent=0
  MOV : powerlib/Elements/Surge Arrester  ProtectionVoltage=152  Columns=30  ReferenceCurrent=50  Segment1=[.955 50]  Segment2=[1.0 25]  Segment3=[.9915 16.5]  Measurements=None  BreakLoop=on
      settings: AttributesFormatString=\n  SourceProductName=Simscape Power Systems  SourceProductBaseCode=PS
  RL Damp. : powerlib/Elements/Parallel RLC Branch  LConnTagsString=a  RConnTagsString=__new0  BranchType=RL  Resistance=7.5  Inductance=1.7e-3  SetiL0=off  InitialCurrent=0  Capacitance=1.0  Setx0=off  InitialVoltage=0  Measurements=None
  UCsa : powerlib/Measurements/Voltage Measurement  Tag=PoWeRsYsTeMmEaSuReMeNt  PhasorSimulation=off  OutputType=Magnitude  PSBequivalent=0
  in : PMIOPort  Side=Left
  "out " : PMIOPort  Port=2  Side=Right
  wires:
  IMOV/1 -> Energy & Gap firing/1(I_MOV)
  UCsa/1 -> Energy & Gap firing/2(U_MOV)
  Energy & Gap firing/1(Gap_trip) -> Gap/1
  connections:
  MOV/RConn1 -- IMOV/LConn1
  RL Damp./LConn1 -- MOV/LConn1 -- Cs/LConn1 -- UCsa/LConn1 -- in/RConn1
  RL Damp./RConn1 -- Gap/LConn1
  IMOV/RConn1 -- Gap/RConn1 -- Cs/RConn1 -- UCsa/LConn2 -- "out "/RConn1

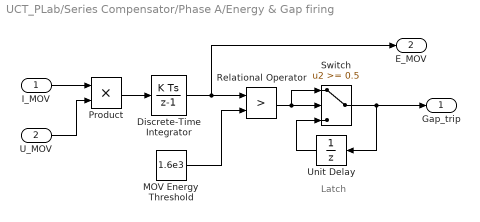
== system UCT_PLab/Series Compensator/Phase A/Energy & Gap firing ==
  note: Latch
  I_MOV : Inport
  U_MOV : Inport  Port=2
  Discrete-Time Integrator : DiscreteIntegrator  SampleTime=-1  ICPrevOutput=DiscIntNeverNeededParam  ICPrevScaledInput=DiscIntNeverNeededParam
  MOV Energy Threshold : Constant  Value=1.6e3
  Product : Product  SaturateOnIntegerOverflow=on  InputSameDT=on  OutDataTypeStr=Inherit: Same as first input
  Relational Operator : RelationalOperator  Operator=>  ZeroCross=off  RndMeth=Nearest  InputSameDT=on
  Switch : Switch  Threshold=0.5  ZeroCross=off  InputSameDT=on
  Unit Delay : UnitDelay  SampleTime=-1
  Gap_trip : Outport
  E_MOV : Outport  Port=2  InitialOutput=0
  wires:
  Switch/1 -> Unit Delay/1, Gap_trip/1
  U_MOV/1 -> Product/2
  MOV Energy Threshold/1 -> Relational Operator/2
  Product/1 -> Discrete-Time Integrator/1
  I_MOV/1 -> Product/1
  Discrete-Time Integrator/1 -> E_MOV/1, Relational Operator/1
  Relational Operator/1 -> Switch/1, Switch/2
  Unit Delay/1 -> Switch/3

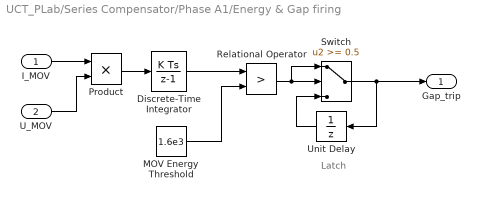
== system UCT_PLab/Series Compensator/Phase A1/Energy & Gap firing ==
  note: Latch
  I_MOV : Inport
  U_MOV : Inport  Port=2
  Discrete-Time Integrator : DiscreteIntegrator  SampleTime=-1  ICPrevOutput=DiscIntNeverNeededParam  ICPrevScaledInput=DiscIntNeverNeededParam
  MOV Energy Threshold : Constant  Value=1.6e3
  Product : Product  SaturateOnIntegerOverflow=on  InputSameDT=on  OutDataTypeStr=Inherit: Same as first input
  Relational Operator : RelationalOperator  Operator=>  ZeroCross=off  RndMeth=Nearest  InputSameDT=on
  Switch : Switch  Threshold=0.5  ZeroCross=off  InputSameDT=on
  Unit Delay : UnitDelay  SampleTime=-1
  Gap_trip : Outport
  wires:
  Unit Delay/1 -> Switch/3
  Relational Operator/1 -> Switch/2, Switch/1
  Discrete-Time Integrator/1 -> Relational Operator/1
  I_MOV/1 -> Product/1
  Product/1 -> Discrete-Time Integrator/1
  MOV Energy Threshold/1 -> Relational Operator/2
  U_MOV/1 -> Product/2
  Switch/1 -> Gap_trip/1, Unit Delay/1

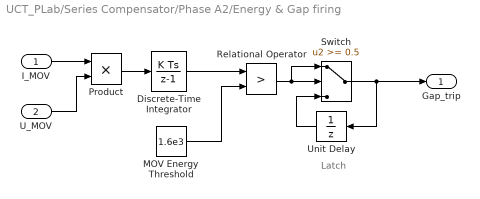
== system UCT_PLab/Series Compensator/Phase A2/Energy & Gap firing ==
  note: Latch
  I_MOV : Inport
  U_MOV : Inport  Port=2
  Discrete-Time Integrator : DiscreteIntegrator  SampleTime=-1  ICPrevOutput=DiscIntNeverNeededParam  ICPrevScaledInput=DiscIntNeverNeededParam
  MOV Energy Threshold : Constant  Value=1.6e3
  Product : Product  SaturateOnIntegerOverflow=on  InputSameDT=on  OutDataTypeStr=Inherit: Same as first input
  Relational Operator : RelationalOperator  Operator=>  ZeroCross=off  RndMeth=Nearest  InputSameDT=on
  Switch : Switch  Threshold=0.5  ZeroCross=off  InputSameDT=on
  Unit Delay : UnitDelay  SampleTime=-1
  Gap_trip : Outport
  wires:
  Switch/1 -> Unit Delay/1, Gap_trip/1
  U_MOV/1 -> Product/2
  MOV Energy Threshold/1 -> Relational Operator/2
  Product/1 -> Discrete-Time Integrator/1
  I_MOV/1 -> Product/1
  Discrete-Time Integrator/1 -> Relational Operator/1
  Relational Operator/1 -> Switch/1, Switch/2
  Unit Delay/1 -> Switch/3

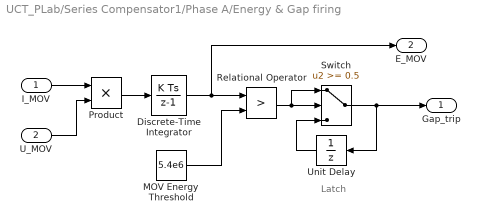
== system UCT_PLab/Series Compensator1/Phase A/Energy & Gap firing ==
  note: Latch
  I_MOV : Inport
  U_MOV : Inport  Port=2
  Discrete-Time Integrator : DiscreteIntegrator  SampleTime=-1  ICPrevOutput=DiscIntNeverNeededParam  ICPrevScaledInput=DiscIntNeverNeededParam
  MOV Energy Threshold : Constant  Value=5.4e6
  Product : Product  SaturateOnIntegerOverflow=on  InputSameDT=on  OutDataTypeStr=Inherit: Same as first input
  Relational Operator : RelationalOperator  Operator=>  ZeroCross=off  RndMeth=Nearest  InputSameDT=on
  Switch : Switch  Threshold=0.5  ZeroCross=off  InputSameDT=on
  Unit Delay : UnitDelay  SampleTime=-1
  Gap_trip : Outport
  E_MOV : Outport  Port=2  InitialOutput=0
  wires:
  Switch/1 -> Unit Delay/1, Gap_trip/1
  U_MOV/1 -> Product/2
  MOV Energy Threshold/1 -> Relational Operator/2
  Product/1 -> Discrete-Time Integrator/1
  I_MOV/1 -> Product/1
  Discrete-Time Integrator/1 -> E_MOV/1, Relational Operator/1
  Relational Operator/1 -> Switch/1, Switch/2
  Unit Delay/1 -> Switch/3

== system UCT_PLab/Series Compensator1/Phase A1/Energy & Gap firing ==
  note: Latch
  I_MOV : Inport
  U_MOV : Inport  Port=2
  Discrete-Time Integrator : DiscreteIntegrator  SampleTime=-1  ICPrevOutput=DiscIntNeverNeededParam  ICPrevScaledInput=DiscIntNeverNeededParam
  MOV Energy Threshold : Constant  Value=5.4e6
  Product : Product  SaturateOnIntegerOverflow=on  InputSameDT=on  OutDataTypeStr=Inherit: Same as first input
  Relational Operator : RelationalOperator  Operator=>  ZeroCross=off  RndMeth=Nearest  InputSameDT=on
  Switch : Switch  Threshold=0.5  ZeroCross=off  InputSameDT=on
  Unit Delay : UnitDelay  SampleTime=-1
  Gap_trip : Outport
  wires:
  Unit Delay/1 -> Switch/3
  Relational Operator/1 -> Switch/2, Switch/1
  Discrete-Time Integrator/1 -> Relational Operator/1
  I_MOV/1 -> Product/1
  Product/1 -> Discrete-Time Integrator/1
  MOV Energy Threshold/1 -> Relational Operator/2
  U_MOV/1 -> Product/2
  Switch/1 -> Gap_trip/1, Unit Delay/1

== system UCT_PLab/Series Compensator1/Phase A2/Energy & Gap firing ==
  note: Latch
  I_MOV : Inport
  U_MOV : Inport  Port=2
  Discrete-Time Integrator : DiscreteIntegrator  SampleTime=-1  ICPrevOutput=DiscIntNeverNeededParam  ICPrevScaledInput=DiscIntNeverNeededParam
  MOV Energy Threshold : Constant  Value=1.5e3
  Product : Product  SaturateOnIntegerOverflow=on  InputSameDT=on  OutDataTypeStr=Inherit: Same as first input
  Relational Operator : RelationalOperator  Operator=>  ZeroCross=off  RndMeth=Nearest  InputSameDT=on
  Switch : Switch  Threshold=0.5  ZeroCross=off  InputSameDT=on
  Unit Delay : UnitDelay  SampleTime=-1
  Gap_trip : Outport
  wires:
  Switch/1 -> Unit Delay/1, Gap_trip/1
  U_MOV/1 -> Product/2
  MOV Energy Threshold/1 -> Relational Operator/2
  Product/1 -> Discrete-Time Integrator/1
  I_MOV/1 -> Product/1
  Discrete-Time Integrator/1 -> Relational Operator/1
  Relational Operator/1 -> Switch/1, Switch/2
  Unit Delay/1 -> Switch/3
